simulink model "master_task"  (Simulink 3.00)
libraries: mathlib x4, inoutlib x4

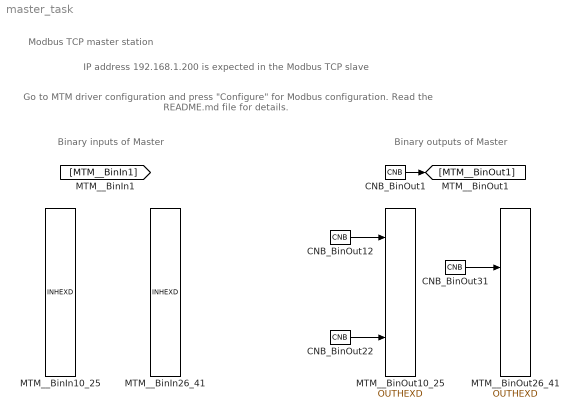
== system master_task ==
  note: Binary inputs of Master
  note: Binary outputs of Master
  note: Modbus TCP master station
  note: IP address 192.168.1.200 is expected in the Modbus TCP slave
  note: Go to MTM driver configuration and press "Configure" for Modbus configuration.
      |
      | Read the README.md file for details.
  CNB_BinOut{1,12,22,31} (4 alike) : mathlib/CNB  YCN=on
  MTM__BinIn10_25 : inoutlib/INHEXD
  MTM__BinIn26_41 : inoutlib/INHEXD
  MTM__BinOut10_25 : inoutlib/OUTHEXD
  MTM__BinOut26_41 : inoutlib/OUTHEXD
  wires:
  CNB_BinOut1/1 -> [MTM__BinOut1]
  CNB_BinOut12/1 -> MTM__BinOut10_25/3
  CNB_BinOut22/1 -> MTM__BinOut10_25/13
  CNB_BinOut31/1 -> MTM__BinOut26_41/6
